simulink model "hw3ece316_p1_2"  (R2018a)
settings: Solver=VariableStepAuto  StartTime=0.0  StopTime=25  RelTol=1e-3
settings Model: Creator=abrun  LastModifiedBy=abrun

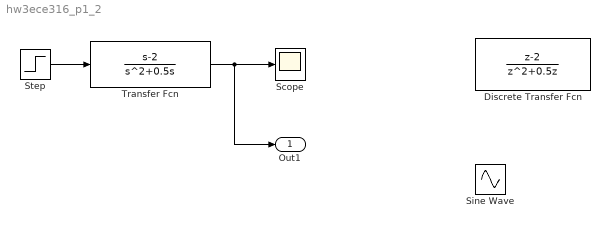
== system hw3ece316_p1_2 ==
  Discrete Transfer Fcn : DiscreteTransferFcn  Numerator=[1 -2]  Denominator=[1 0.5 0]
  Scope : Scope
  Sine Wave : Sin  SampleTime=0
  Step : Step  SampleTime=0
  Transfer Fcn : TransferFcn  Numerator=[1 -2]  Denominator=[1 0.5 0]
  Out1 : Outport  SignalName=y
  wires:
  Transfer Fcn/1 -> Out1/1, Scope/1
  Step/1 -> Transfer Fcn/1
